simulink model "TrafficLightController"  (R2020b)
settings: Solver=VariableStepAuto  StartTime=0.0  StopTime=10.0  RelTol=1e-3
undefined symbols (not defined in the file): DiscIntNeverNeededParam
libraries: simulink x1
settings Model: Creator=BIDITA PAUL  LastModifiedBy=BIDITA PAUL

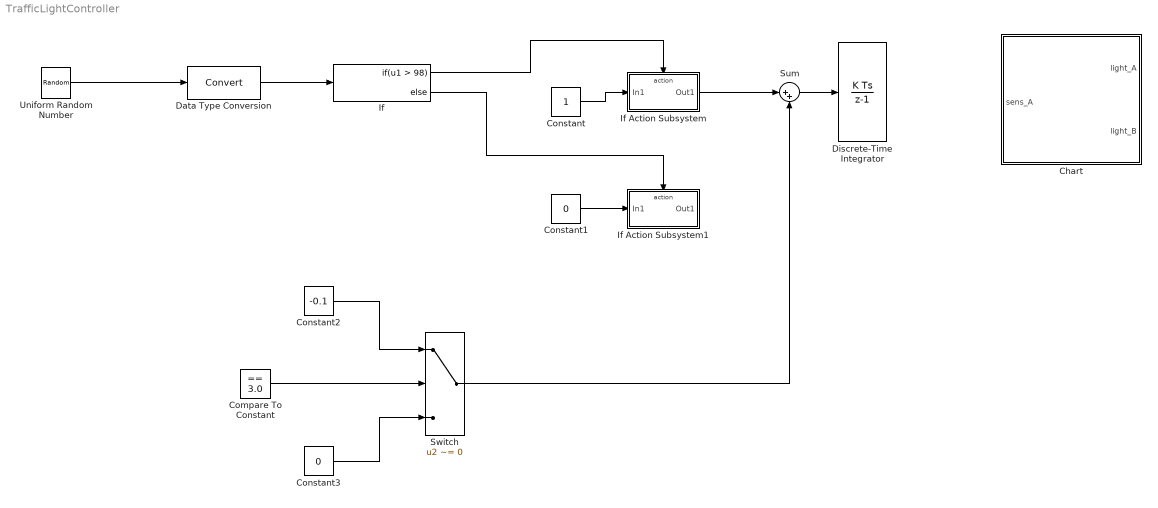
== system TrafficLightController ==
  Chart : Stateflow chart  TreatAsAtomicUnit=on
  Compare To Constant : simulink/Logic and Bit Operations/Compare To Constant  relop===  const=3.0  OutDataTypeStr=boolean
  Constant : Constant
  Constant1 : Constant  Value=0
  Constant2 : Constant  Value=-0.1
  Constant3 : Constant  Value=0
  Data Type Conversion : DataTypeConversion
  Discrete-Time Integrator : DiscreteIntegrator  SampleTime=-1  LimitOutput=on  LowerSaturationLimit=0  ICPrevOutput=DiscIntNeverNeededParam  ICPrevScaledInput=DiscIntNeverNeededParam
  If : If  IfExpression=u1 > 98
  If Action Subsystem : Subsystem  TreatAsAtomicUnit=on
  If Action Subsystem1 : Subsystem  TreatAsAtomicUnit=on
  Sum : Sum  Inputs=|++
  Switch : Switch  Criteria=u2 ~= 0
  Uniform Random Number : UniformRandomNumber  Minimum=0  Maximum=100  Seed=177836  SampleTime=0
  wires:
  Data Type Conversion/1 -> If/1
  Uniform Random Number/1 -> Data Type Conversion/1
  If/1 -> If Action Subsystem/Action
  If/2 -> If Action Subsystem1/Action
  Constant/1 -> If Action Subsystem/1(In1)
  Constant1/1 -> If Action Subsystem1/1(In1)
  Compare To Constant/1 -> Switch/2
  Switch/1 -> Sum/2
  If Action Subsystem/1(Out1) -> Sum/1
  Constant2/1 -> Switch/1
  Constant3/1 -> Switch/3
  Sum/1 -> Discrete-Time Integrator/1

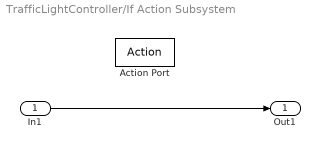
== system TrafficLightController/If Action Subsystem ==
  In1 : Inport
  Action Port : ActionPort  ActionPortLabel=if(u1 > 0)
  Out1 : Outport
  wires:
  In1/1 -> Out1/1

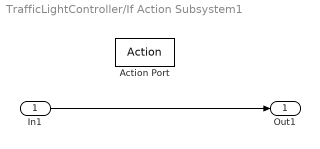
== system TrafficLightController/If Action Subsystem1 ==
  In1 : Inport
  Action Port : ActionPort  ActionPortLabel=else
  Out1 : Outport
  wires:
  In1/1 -> Out1/1

== stateflow chart TrafficLightController/Chart ==
  state S0
    entry:
    light_A =2;
    light_B = 0;
  state S1
    entry:
    light_A = 2;
    light_B = 0;
  state S2
    entry:
    light_A = 1;
    light_B = 0;
  state S4
    entry:
    light_A = 0;
    light_B = 1;
  state S3
    entry:
    light_A = 0;
    light_B = 2;
  (default) -> S0
  S0 -> S1 : after(30,tick)
  S1 -> S2 : [sens_A]
  S4 -> S0 : after(3,tick)
  S2 -> S3 : after(3,tick)
  S3 -> S4 : after(10,tick)
  data: sens_A input; light_A output; light_B output
